simulink model "planLocal_ros"  (R2024a)
settings: Solver=FixedStepDiscrete  StartTime=0.0  StopTime=30  RelTol=1e-3
InitFcn:
  | % Make sure server is running
  | svrMdlName = 'localPlanServer';
  | load_system(svrMdlName);
  | set_param(svrMdlName,'SimulationCommand','Start');
  | pause(1);
StopFcn:
  | % Make sure server is running
  | svrMdlName = 'localPlanServer';
  | load_system(svrMdlName);
  | set_param(svrMdlName,'SimulationCommand','Stop');
undefined symbols (not defined in the file): costweights, curpose, curvel, gridloc, lastidx, lookaheadtime, mat, maxacceleration, maxreversevelocity, maxvelocity, minturningradius, n, obstaclesafetymargin, refPath, refpath, resolution, tuneabletebparams, tuneableTEBParamsCpp, worldGridLoc, worldMat, worldRes
libraries: roshelperlib x8, ros2lib x2, simulink x1
settings Model: Creator=cstabile  LastModifiedBy=cstabile
settings SFSimCC: SimTargetLang=C++

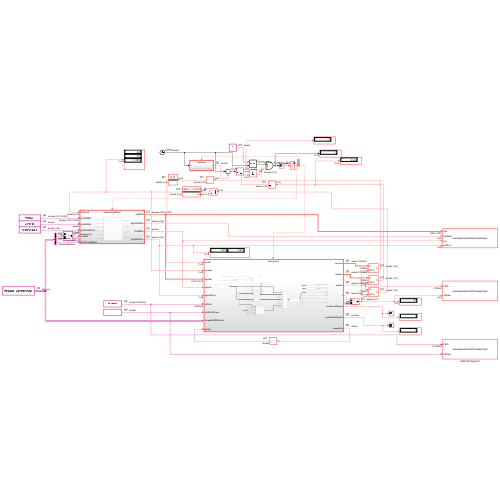
[thumbnail: Simulink's stored preview of the top-level diagram]
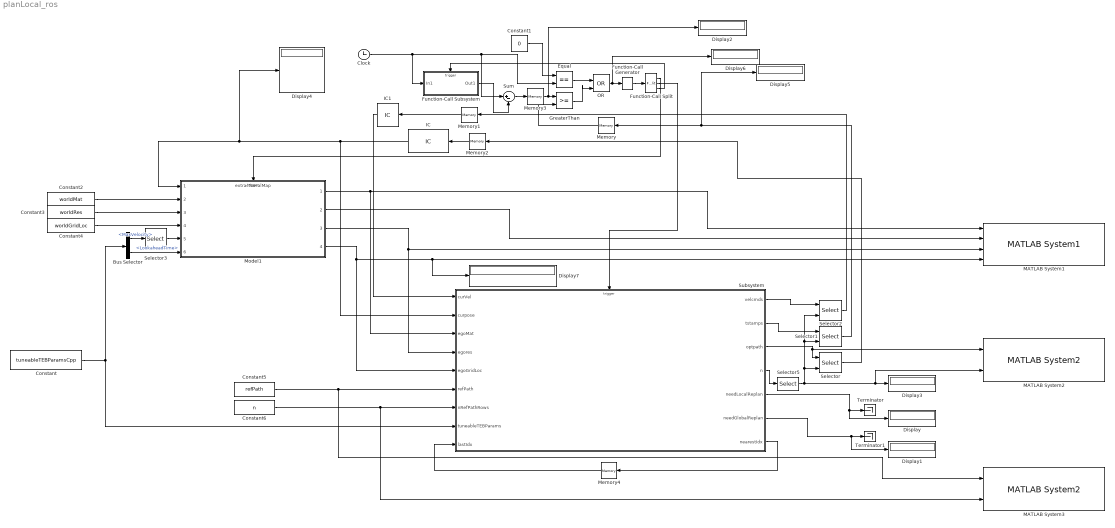
== system planLocal_ros ==
  Bus Selector : BusSelector  OutputSignals=MaxVelocity,LookaheadTime
  Clock : Clock
  Constant : Constant  Value=tuneableTEBParamsCpp  OutDataTypeStr=Bus: teb_bus
  Constant1 : Constant  Value=0
  Constant2 : Constant  Value=worldMat  VectorParams1D=off
  Constant3 : Constant  Value=worldRes
  Constant4 : Constant  Value=worldGridLoc  VectorParams1D=off
  Constant5 : Constant  Value=refPath  VectorParams1D=off
  Constant6 : Constant  Value=n
  Display{,1..7} (8 alike) : Display
  Equal : RelationalOperator  Operator===  OutDataTypeStr=boolean  RndMeth=Simplest  InputSameDT=off
  Function-Call Generator : simulink/Ports & Subsystems/Function-Call Generator  sample_time=1  numberOfIterations=1  DisallowWideOutput=off  ShowEnablePort=on
  Function-Call Split : FunctionCallSplit  IconShape=distinctive  NumOutputPorts=3  OutputPortLayout=default
  Function-Call Subsystem : Subsystem  TreatAsAtomicUnit=on
  GreaterThan : RelationalOperator  OutDataTypeStr=boolean  RndMeth=Simplest  InputSameDT=off
  IC : InitialCondition  Value=refPath(1,:) + [10 10 0]
  IC1 : InitialCondition  Value=[0 0]
  MATLAB System1 : roshelperlib/MATLAB System1  MapType=SDF  IsEgo=off  DisplayVisual=on  SimulateUsing=Interpreted execution
  MATLAB System2 : roshelperlib/MATLAB System2  VisualizationParameters={'k-'}  PlotType=Line  DisplayVisual=on  SimulateUsing=Interpreted execution
  MATLAB System3 : roshelperlib/MATLAB System2  VisualizationParameters={'r:','LineWidth',5}  PlotType=Line  DisplayVisual=on  SimulateUsing=Interpreted execution
  Memory{,1..4} (5 alike) : Memory
  Model1 : ModelReference  ModelNameDialog=extractLocalMap.slx  SimulationMode=Normal  ModelReferenceVersion=1.0  TriggerPortName=function  TriggerPortTriggerType=function-call  TriggerPortStatesWhenEnabling=held
  OR : Logic  Operator=OR  IconShape=distinctive  AllPortsSameDT=off  OutDataTypeStr=boolean
  Selector : Selector  NumberOfDimensions=2  InputPortWidth=3  IndexOptions=Index vector (port),Select all  Indices=[1 3],1  OutputSizes=1,1
  Selector1 : Selector  NumberOfDimensions=2  InputPortWidth=3  IndexOptions=Index vector (port),Index vector (dialog)  Indices=[1 3],1  OutputSizes=1,1
  Selector2 : Selector  NumberOfDimensions=2  InputPortWidth=3  IndexOptions=Index vector (port),Index vector (dialog)  Indices=[1 3],[1 2]  OutputSizes=1,1
  Selector3 : Selector  InputPortWidth=2  IndexOptions=Index vector (dialog)  Indices=1  OutputSizes=1
  Selector5 : Selector  InputPortWidth=2  IndexOptions=Index vector (dialog)  Indices=1  OutputSizes=1
  Subsystem : Subsystem
  Sum : Sum  Inputs=|+-
  Terminator : Terminator
  Terminator1 : Terminator
  wires:
  Clock/1 -> Function-Call Subsystem/1(In1), Sum/1, Equal/2
  GreaterThan/1 -> OR/2
  Equal/1 -> OR/1
  Constant1/1 -> Equal/1
  OR/1 -> Display6/1, Function-Call Generator/1
  Selector/1 -> Memory2/1
  Constant2/1 -> Model1/2
  Constant3/1 -> Model1/3
  Constant4/1 -> Model1/4
  Bus Selector/2 -> Model1/6  "<LookaheadTime>"
  Bus Selector/1 -> Selector3/1  "<MaxVelocity>"
  Model1/4 -> Display7/1, MATLAB System1/4, Subsystem/5(egoGridLoc)
  Constant/1 -> Subsystem/8(tuneableTEBParams), Bus Selector/1
  Model1/3 -> MATLAB System1/3, Subsystem/4(egores)
  Model1/2 -> MATLAB System1/2
  Model1/1 -> Subsystem/3(egoMat), MATLAB System1/1
  Function-Call Split/2 -> Subsystem/Trigger
  IC/1 -> Model1/1, Display4/1, Subsystem/2(curpose)
  Selector3/1 -> Model1/5
  Function-Call Generator/1 -> Function-Call Split/1
  Function-Call Split/1 -> Model1/Trigger
  Memory/1 -> GreaterThan/2
  Memory1/1 -> IC1/1
  Memory2/1 -> IC/1
  Function-Call Split/3 -> Function-Call Subsystem/Trigger
  Function-Call Subsystem/1(Out1) -> Sum/2
  Sum/1 -> Memory3/1
  Memory3/1 -> Display2/1, GreaterThan/1
  Subsystem/4(n) -> Selector5/1
  Selector1/1 -> Display5/1, Memory/1
  Subsystem/3(optpath) -> MATLAB System2/1, Selector/1
  Subsystem/5(needLocalReplan) -> Display/1, Terminator/1
  Subsystem/6(needGlobalReplan) -> Display1/1, Terminator1/1
  IC1/1 -> Subsystem/1(curVel)
  Constant5/1 -> MATLAB System3/1, Subsystem/6(refPath)
  Constant6/1 -> MATLAB System3/2, Subsystem/7(nRefPathRows)
  Selector2/1 -> Memory1/1
  Subsystem/2(tstamps) -> Selector1/1
  Subsystem/1(velcmds) -> Selector2/1
  Selector5/1 -> MATLAB System2/2, Display3/1, Selector/2, Selector2/2, Selector1/2
  Subsystem/7(nearestIdx) -> Memory4/1
  Memory4/1 -> Subsystem/9(lastIdx)

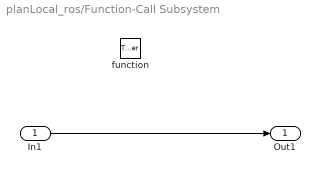
== system planLocal_ros/Function-Call Subsystem ==
  In1 : Inport
  function : TriggerPort  TriggerType=function-call  VariantControl=(inherit)
  Out1 : Outport
  wires:
  In1/1 -> Out1/1

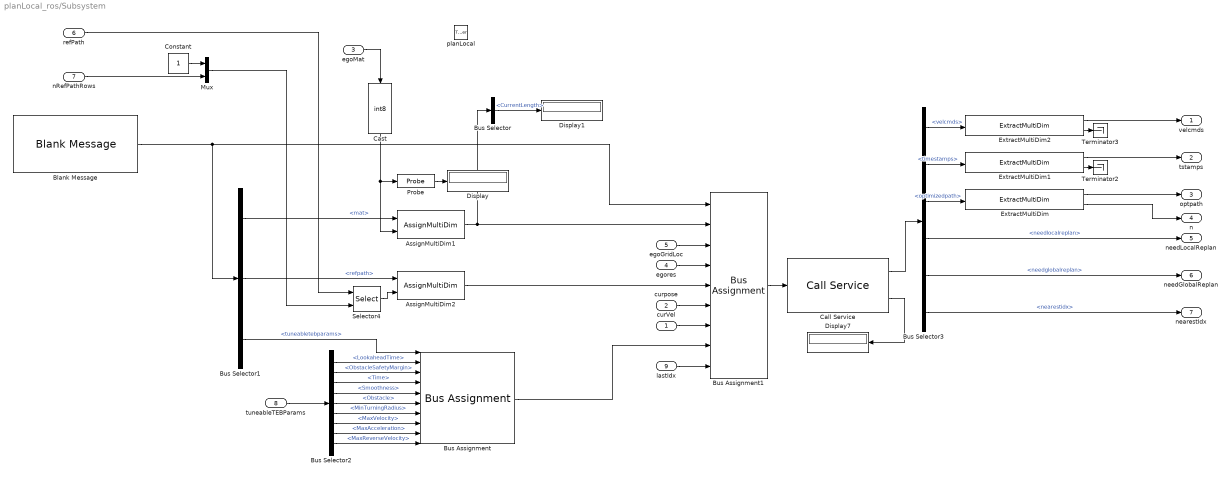
== system planLocal_ros/Subsystem ==
  curVel : Inport
  curpose : Inport  Port=2
  egoMat : Inport  Port=3
  egores : Inport  Port=4
  egoGridLoc : Inport  Port=5
  refPath : Inport  Port=6
  nRefPathRows : Inport  Port=7
  tuneableTEBParams : Inport  Port=8
  lastIdx : Inport  Port=9
  planLocal : TriggerPort  TriggerType=function-call  VariantControl=(inherit)
  AssignMultiDim1 : roshelperlib/AssignMultiDim  SystemSampleTime=-1  VariantActivationTime=update diagram  AllowFlexibleInterface=on  Latency=0  AutoFrameSizeCalculation=off
  AssignMultiDim2 : roshelperlib/AssignMultiDim  SystemSampleTime=-1  VariantActivationTime=update diagram  AllowFlexibleInterface=on  Latency=0  AutoFrameSizeCalculation=off
  Blank Message : ros2lib/Blank Message  messageClass=Service Request  entityType=offroad_msg/PlanLocal  messageType=offroad_msg/PlanLocalRequest  SampleTime=inf
  Bus Assignment : BusAssignment  AssignedSignals=lookaheadtime,obstaclesafetymargin,costweights.time,costweights.smoothness,costweights.obstacle,minturningradius,maxvelocity,maxacceleration,maxreversevelocity
  Bus Assignment1 : BusAssignment  AssignedSignals=mat,gridloc,resolution,refpath,curpose,curvel,tuneabletebparams,lastidx
  Bus Selector : BusSelector  OutputSignals=data_SL_Info.CurrentLength
  Bus Selector1 : BusSelector  OutputSignals=mat,refpath,tuneabletebparams
  Bus Selector2 : BusSelector  OutputSignals=LookaheadTime,ObstacleSafetyMargin,CostWeights_T.Time,CostWeights_T.Smoothness,CostWeights_T.Obstacle,MinTurningRadius,MaxVelocity,MaxAcceleration,MaxReverseVelocity
  Bus Selector3 : BusSelector  OutputSignals=velcmds,timestamps,optimizedpath,needlocalreplan,needglobalreplan,nearestidx
  Call Service : ros2lib/Call Service  topicSource=Specify your own  service=/planLocal  serviceType=offroad_msg/PlanLocal  connectionTimeout=5  ShowErrorCodeOutput=on  legacyBusStruct=off  QOSHistory=Keep last  QOSDepth=1  QOSReliability=Reliable  QOSDurability=Volatile  QOSDeadline=Inf  QOSLifespan=Inf  QOSLiveliness=Automatic  QOSLeaseDuration=Inf  QOSAvoidROSNamespaceConventions=off
  Cast : DataTypeConversion  OutDataTypeStr=int8  SaturateOnIntegerOverflow=off  RndMeth=Floor
  Constant : Constant
  Display : Display
  Display1 : Display
  Display7 : Display
  ExtractMultiDim : roshelperlib/ExtractMultiDim  userDataType=double  dims=[1000 3]  isVarsize=on  varsizeDims=[1 0]  returnFixedTF=on
  ExtractMultiDim1 : roshelperlib/ExtractMultiDim  userDataType=double  dims=[1000 1]  isVarsize=on  varsizeDims=[1 0]  returnFixedTF=off
  ExtractMultiDim2 : roshelperlib/ExtractMultiDim  userDataType=double  dims=[1000 2]  isVarsize=on  varsizeDims=[1 0]  returnFixedTF=off
  Mux : Mux  Inputs=2
  Probe : Probe  ProbeWidth=off  ProbeSampleTime=off  ProbeComplexSignal=off  ProbeSignalDimensions=on
  Selector4 : Selector  NumberOfDimensions=2  IndexMode=Zero-based  InputPortWidth=3  IndexOptions=Starting and ending indices (port),Select all  Indices=[1 3],1  OutputSizes=1,1
  Terminator2 : Terminator
  Terminator3 : Terminator
  velcmds : Outport
  tstamps : Outport  Port=2
  optpath : Outport  Port=3
  n : Outport  Port=4
  needLocalReplan : Outport  Port=5
  needGlobalReplan : Outport  Port=6
  nearestIdx : Outport  Port=7
  wires:
  Bus Selector3/3 -> ExtractMultiDim/1  "<optimizedpath>"
  AssignMultiDim2/1 -> Bus Assignment1/5
  Bus Selector2/6 -> Bus Assignment/7  "<MinTurningRadius>"
  Bus Selector1/1 -> AssignMultiDim1/1  "<mat>"
  Cast/1 -> Probe/1, AssignMultiDim1/2
  Bus Assignment1/1 -> Call Service/1
  Blank Message/1 -> Bus Selector1/1, Bus Assignment1/1
  Bus Selector3/4 -> needLocalReplan/1  "<needlocalreplan>"
  AssignMultiDim1/1 -> Bus Assignment1/2, Bus Selector/1
  Bus Selector3/2 -> ExtractMultiDim1/1  "<timestamps>"
  Bus Selector3/5 -> needGlobalReplan/1  "<needglobalreplan>"
  Call Service/2 -> Display7/1
  ExtractMultiDim1/2 -> Terminator2/1
  Bus Selector2/2 -> Bus Assignment/3  "<ObstacleSafetyMargin>"
  Call Service/1 -> Bus Selector3/1
  Bus Selector1/3 -> Bus Assignment/1  "<tuneabletebparams>"
  egores/1 -> Bus Assignment1/4
  Bus Selector2/4 -> Bus Assignment/5  "<Smoothness>"
  ExtractMultiDim1/1 -> tstamps/1
  Bus Selector2/9 -> Bus Assignment/10  "<MaxReverseVelocity>"
  Selector4/1 -> AssignMultiDim2/2
  Bus Selector1/2 -> AssignMultiDim2/1  "<refpath>"
  Bus Selector2/1 -> Bus Assignment/2  "<LookaheadTime>"
  Bus Selector2/3 -> Bus Assignment/4  "<Time>"
  nRefPathRows/1 -> Mux/2
  Bus Selector2/7 -> Bus Assignment/8  "<MaxVelocity>"
  ExtractMultiDim2/1 -> velcmds/1
  ExtractMultiDim/1 -> optpath/1
  Bus Selector2/5 -> Bus Assignment/6  "<Obstacle>"
  refPath/1 -> Selector4/1
  Bus Selector2/8 -> Bus Assignment/9  "<MaxAcceleration>"
  ExtractMultiDim2/2 -> Terminator3/1
  Bus Selector3/1 -> ExtractMultiDim2/1  "<velcmds>"
  tuneableTEBParams/1 -> Bus Selector2/1
  egoMat/1 -> Cast/1
  ExtractMultiDim/2 -> n/1
  Constant/1 -> Mux/1
  Mux/1 -> Selector4/2
  Probe/1 -> Display/1
  Bus Selector/1 -> Display1/1  "<CurrentLength>"
  egoGridLoc/1 -> Bus Assignment1/3
  curpose/1 -> Bus Assignment1/6
  curVel/1 -> Bus Assignment1/7
  Bus Assignment/1 -> Bus Assignment1/8
  Bus Selector3/6 -> nearestIdx/1  "<nearestidx>"
  lastIdx/1 -> Bus Assignment1/9
